simulink model "angleClosedloop_hw"  (R2020a)
settings: Solver=FixedStepAuto  StartTime=0.0  StopTime=30  FixedStep=TS  RelTol=1e-3  EnableMultiTasking=on
PostLoadFcn:
  | paramsBasicKinematics
  | load('MotorResponse.mat')
model workspace (MAT data in the model file):
  TS = 0.01
undefined symbols (not defined in the file): L, PWMcmdMono_L, PWMcmdMono_R, r, sigbuilder_block, speedMono_L, speedMono_R
libraries: arduinomotorcarrierlib x4, simulink_extras x4, simulink x1
settings Model: SimulationMode=external  SILPILModeSetting=veronly  ExtModeTrigDuration=2  Creator=jmodiset  LastModifiedBy=mmarathe
settings DataIOCC: ReturnWorkspaceOutputs=off
settings OptimizationCC: PassReuseOutputArgsThreshold=0  MaxStackSize=64
settings DebuggingCC: ParameterTunabilityLossMsg=error  PregeneratedLibrarySubsystemCodeDiagnostic=none  ArithmeticOperatorsInVariantConditions=warning
settings HardwareCC: ProdBitPerPointer=32  ProdBitPerSizeT=32  ProdBitPerPtrDiffT=32  ProdLargestAtomicInteger=Long  ProdLargestAtomicFloat=Double  ProdWordSize=32  ProdHWDeviceType=ARM Compatible->ARM Cortex
settings SFSimCC: SimUseLocalCustomCode=off  MATLABDynamicMemAlloc=off  CustomCodeUndefinedFunction=UseInterfaceOnly
settings RTWCC: SystemTargetFile=ert.tlc  HardwareBoard=Arduino Nano 33 IoT  TLCOptions=-aInlineSetEventsForThisBaseRateFcn=TLC_FALSE -aSuppressMultiTaskScheduler=TLC_FALSE -aRateBasedStepFcn=1  TemplateMakefile=ert_default_tmf  RTWUseLocalCustomCode=off  Toolchain=Arduino ARM  BuildConfiguration=Faster Runs
settings CodeAppCC: ForceParamTrailComments=on  OperatorAnnotations=on
settings ERTTargetCC: ERTCustomFileBanners=off  SupportContinuousTime=on  SupportNonInlinedSFcns=on  RemoveResetFunc=off  SupportVariableSizeSignals=on  ModelStepFunctionPrototypeControlCompliant=off  ExtModeStaticAllocSize=8192

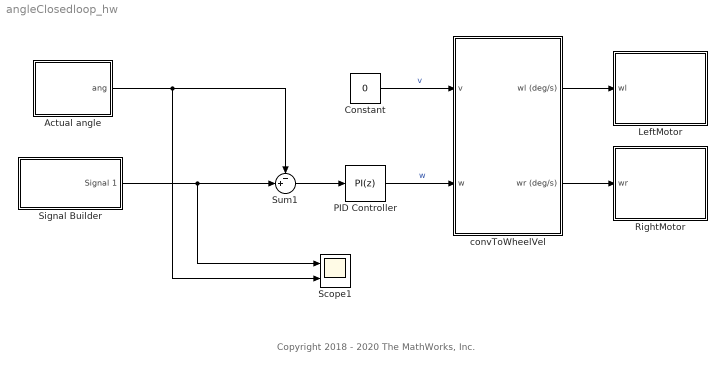
== system angleClosedloop_hw ==
  note: Copyright 2018 - 2020 The MathWorks, Inc.
  Actual angle : Subsystem
  Constant : Constant  Value=0
  LeftMotor : Subsystem
      mask Display:
      | color('white');
      | plot([100,100,100,100]*1,[100,100,100,100]*1);
      | plot([100,100,100,100]*0,[100,100,100,100]*0);
      | sppkgroot = strrep(codertarget.arduinobase.internal.getBaseSpPkgRootDir(),'\','/');
      | image(fullfile(sppkgroot,'resources','dcmotor.png'),'center')
  "PID Controller " : simulink/Continuous/PID Controller  Controller=PI  Form=Parallel  TimeDomain=Discrete-time  UseExternalTs=off  SampleTime=-1  IntegratorMethod=Forward Euler  FilterMethod=Forward Euler  ControllerParametersSource=internal  P=3  I=1  D=0  UseFilter=on  N=100  TunerSelectOption=Transfer Function Based (PID Tuner App)  InitialConditionSource=internal  InitialConditionForIntegrator=0  InitialConditionForFilter=0  DifferentiatorICPrevScaledInput=0  ExternalReset=none  TrackingMode=off  Kt=1  LimitOutput=off  UpperSaturationLimit=inf  LowerSaturationLimit=-inf  LinearizeAsGain=on  AntiWindupMode=none  Kb=1  POutMin=[]  POutMax=[]  IOutMin=[]  IOutMax=[]  DOutMin=[]  DOutMax=[]  NOutMin=[]  NOutMax=[]  SumOutMin=[]  SumOutMax=[]  SaturationOutMin=[]  SaturationOutMax=[]  PParamMin=[]  PParamMax=[]  IParamMin=[]  IParamMax=[]  DParamMin=[]  DParamMax=[]  NParamMin=[]  NParamMax=[]  KbParamMin=[]  KbParamMax=[]  KtParamMin=[]  KtParamMax=[]  KbOutMin=[]  KbOutMax=[]  KtOutMin=[]  KtOutMax=[]  IntegratorOutMin=[]  IntegratorOutMax=[]  FilterOutMin=[]  FilterOutMax=[]  SumI1OutMin=[]  SumI1OutMax=[]  SumI2OutMin=[]  SumI2OutMax=[]  SumI3OutMin=[]  SumI3OutMax=[]  SumI4OutMin=[]  SumI4OutMax=[]  SumDOutMin=[]  SumDOutMax=[]  DifferentiatorOutMin=[]  DifferentiatorOutMax=[]  FilterDiffOutCoefMin=[]  FilterDiffOutCoefMax=[]  ReciprocalOutMin=[]  ReciprocalOutMax=[]  SumDenOutMin=[]  SumDenOutMax=[]  SumNumOutMin=[]  SumNumOutMax=[]  DivideOutMin=[]  DivideOutMax=[]  UdiffTsProdOutMin=[]  UdiffTsProdOutMax=[]  NTsProdOutMin=[]  NTsProdOutMax=[]  UintegralTsProdOutMin=[]  UintegralTsProdOutMax=[]  UngainTsProdOutMin=[]  UngainTsProdOutMax=[]  IntegratorContinuousStateAttributes=''  IntegratorStateMustResolveToSignalObject=off  IntegratorRTWStateStorageClass=Auto  FilterContinuousStateAttributes=''  FilterStateMustResolveToSignalObject=off  FilterRTWStateStorageClass=Auto  ParallelPVariant=InternalParameters  IdealPVariant=Disabled  IVariant=InternalParameters  DVariant=Disabled  IntegratorVariant=Discrete  SatVariant=Disabled  AWVariant=Passthrough  PCopyVariant=Disabled  TRVariant=Disabled  FdbkBlocksVariant=Forward  IdealPFdbkVariant=Disabled  SatFdbkVariant=Disabled  DerivativeFilterVariant=Disabled  NVariant=Disabled  NCopyVariant=Disabled_SignalSpec  FilterICVariant=Disabled  IntegratorICVariant=InternalICs  ExternalResetVariant=Disabled  TRSumVariant=Passthrough  SumFdbkVariant=Disabled  SumVariant=Sum_PI  TsampFilterVariant=InternalTs  TsampNgainVariant=Passthrough  TsampIntegralVariant=Passthrough
  RightMotor : Subsystem
      mask Display:
      | color('white');
      | plot([100,100,100,100]*1,[100,100,100,100]*1);
      | plot([100,100,100,100]*0,[100,100,100,100]*0);
      | sppkgroot = strrep(codertarget.arduinobase.internal.getBaseSpPkgRootDir(),'\','/');
      | image(fullfile(sppkgroot,'resources','dcmotor.png'),'center')
  Scope1 : Scope  NumInputPorts=2
  "Signal Builder " : Subsystem  Tag=STV Subsys  LoadFcn=sigbuilder_block('load');  StartFcn=sigbuilder_block('start');  StopFcn=sigbuilder_block('stop');  ClipboardFcn=sigbuilder_block('clipboard');  mask(Sigbuilder block){tuvar=[0:10]}
      mask help: Simulink:masks:SigbuilderBlock_MD
      mask init:
      | if ~strcmp(get_param(bdroot(gcbh),'SimulationStatus'),'stopped') tuvar = sigbuilder_block('maskInit'); end
      settings: CopyFcn=sigbuilder_block('copy');  DeleteFcn=sigbuilder_block('delete');  ModelCloseFcn=sigbuilder_block('modelClose');  PreSaveFcn=sigbuilder_block('preSave');  PauseFcn=sigbuilder_block('pause');  ContinueFcn=sigbuilder_block('continue');  NameChangeFcn=sigbuilder_block('namechange');  OpenFcn=sigbuilder_block('open',[256.5 124.5 550.5 399.75 ]);  CloseFcn=sigbuilder_block('close');
      mask Display: plot(0, 0, 100, 100,[2, 2, 32, 32, 2], [68, 8, 8, 68, 68],[32, 2], [38, 38], [32, 19, 2],[53, 60, 44], [32, 17, 17, 2],[16, 16, 31, 31]);txt = getActiveGroup(gcbh);text(2, 100, txt,'verticalAlignment', 'top');
  Sum1 : Sum  Inputs=-+|
  convToWheelVel : Subsystem
  wires:
  Actual angle/1(ang) -> Scope1/2, Sum1/1
  Sum1/1 -> "PID Controller "/1
  "Signal Builder "/1(Signal 1) -> Sum1/2, Scope1/1
  Constant/1 -> convToWheelVel/1(v)  "v"
  "PID Controller "/1 -> convToWheelVel/2(w)  "w"
  convToWheelVel/1(wl (deg/s)) -> LeftMotor/1(wl)
  convToWheelVel/2(wr (deg/s)) -> RightMotor/1(wr)

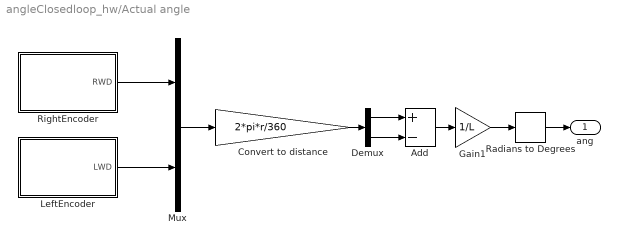
== system angleClosedloop_hw/Actual angle ==
  Add : Sum  Inputs=+-
  Convert to distance : Gain  Gain=2*pi*r/360
  Demux : Demux  Outputs=2
  Gain1 : Gain  Gain=1/L
  LeftEncoder : Subsystem
  Mux : Mux  Inputs=2
  Radians to Degrees : simulink_extras/Transformations/Radians to Degrees
  RightEncoder : Subsystem
  ang : Outport  VectorParamsAs1DForOutWhenUnconnected=off
  wires:
  RightEncoder/1(RWD) -> Mux/1
  Gain1/1 -> Radians to Degrees/1
  Add/1 -> Gain1/1
  Demux/2 -> Add/2
  Convert to distance/1 -> Demux/1
  Demux/1 -> Add/1
  Mux/1 -> Convert to distance/1
  LeftEncoder/1(LWD) -> Mux/2
  Radians to Degrees/1 -> ang/1

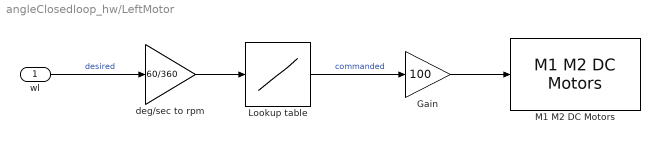
== system angleClosedloop_hw/LeftMotor ==
  wl : Inport
  Gain : Gain  Gain=100
  Lookup table : Lookup_n-D  NumberOfTableDimensions=1  BreakpointsForDimension1=speedMono_L  Table=PWMcmdMono_L  UseLastTableValue=on  InternalRulePriority=Speed  RndMeth=Simplest  InputSameDT=on
  M1 M2 DC Motors : arduinomotorcarrierlib/M1 M2 DC Motors  SlaveAddress=uint8( hex2dec( '66' ) )  blockPlatform=ARDUINO  MotorNumber=M2  MotorCarrierPWMFreq=100
      settings: SourceProductName=Simulink Support Package for Arduino Hardware
  deg/sec to rpm : Gain  Gain=60/360
  wires:
  wl/1 -> deg/sec to rpm/1  "desired"
  Lookup table/1 -> Gain/1  "commanded"
  Gain/1 -> M1 M2 DC Motors/1
  deg/sec to rpm/1 -> Lookup table/1

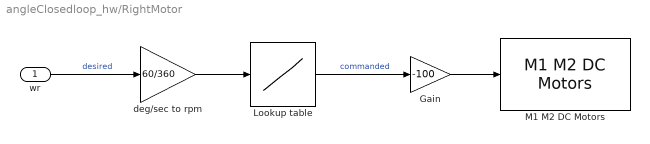
== system angleClosedloop_hw/RightMotor ==
  wr : Inport
  Gain : Gain  Gain=-100
  Lookup table : Lookup_n-D  NumberOfTableDimensions=1  BreakpointsForDimension1=speedMono_R  Table=PWMcmdMono_R  UseLastTableValue=on  InternalRulePriority=Speed  RndMeth=Simplest  InputSameDT=on
  M1 M2 DC Motors : arduinomotorcarrierlib/M1 M2 DC Motors  SlaveAddress=uint8( hex2dec( '66' ) )  blockPlatform=ARDUINO  MotorNumber=M1  MotorCarrierPWMFreq=100
      settings: SourceProductName=Simulink Support Package for Arduino Hardware
  deg/sec to rpm : Gain  Gain=60/360
  wires:
  wr/1 -> deg/sec to rpm/1  "desired"
  Lookup table/1 -> Gain/1  "commanded"
  Gain/1 -> M1 M2 DC Motors/1
  deg/sec to rpm/1 -> Lookup table/1

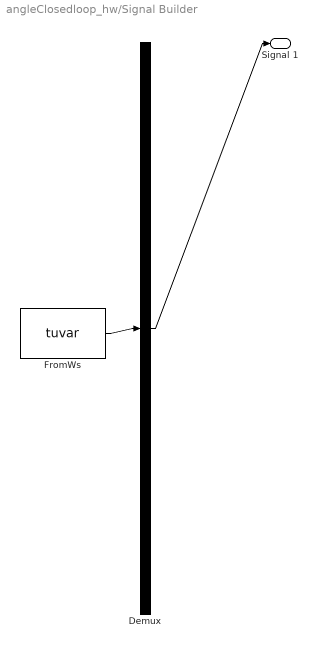
== system angleClosedloop_hw/Signal Builder  ==
  Demux : Demux  Tag=STV Demux  Outputs=1
      settings: DisplayOption=none
  FromWs : FromWorkspace  Tag=STV FromWs  VariableName=tuvar
      SigBuilderData=|
      | common.afterFinalStr = 'Extrapolate'
      | common.sampleTime = 0
      | dataSet.timeRange = [0 30]
      | dataSet.name = 'Group 1'
      | sbobj.Groups.Name = 'Group 1'
      | sbobj.Groups.Signals.Name = 'Signal 1'
      | sbobj.Groups.Signals.XData = [0 5 5 30]
      | sbobj.Groups.Signals.YData = [0 0 90 90]
      | sbobj.Groups.TimeRange = [0 30]
  Signal 1 : Outport  Tag=STV Outport  VectorParamsAs1DForOutWhenUnconnected=off
  wires:
  Demux/1 -> Signal 1/1
  FromWs/1 -> Demux/1

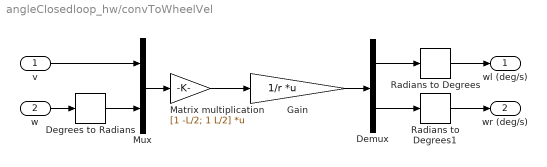
== system angleClosedloop_hw/convToWheelVel ==
  v : Inport
  w : Inport  Port=2
  " Gain" : Gain  Gain=1/r  Multiplication=Matrix(K*u)
  Degrees to Radians : simulink_extras/Transformations/Degrees to Radians
  Demux : Demux  Outputs=2
  Matrix multiplication : Gain  Gain=[1 -L/2; 1 L/2]  Multiplication=Matrix(K*u)
  Mux : Mux  Inputs=2
  Radians to Degrees : simulink_extras/Transformations/Radians to Degrees
  Radians to Degrees1 : simulink_extras/Transformations/Radians to Degrees
  wl (deg/s) : Outport  VectorParamsAs1DForOutWhenUnconnected=off
  wr (deg/s) : Outport  Port=2  VectorParamsAs1DForOutWhenUnconnected=off
  wires:
  " Gain"/1 -> Demux/1
  Matrix multiplication/1 -> " Gain"/1
  v/1 -> Mux/1
  Mux/1 -> Matrix multiplication/1
  Demux/1 -> Radians to Degrees/1
  Demux/2 -> Radians to Degrees1/1
  w/1 -> Degrees to Radians/1
  Radians to Degrees/1 -> wl (deg/s)/1
  Radians to Degrees1/1 -> wr (deg/s)/1
  Degrees to Radians/1 -> Mux/2

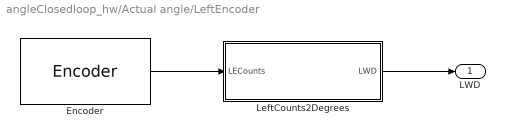
== system angleClosedloop_hw/Actual angle/LeftEncoder ==
  Encoder : arduinomotorcarrierlib/Encoder  SlaveAddress=uint8( hex2dec( '66' ) )  blockPlatform=ARDUINO  Encoder=2  ShowSpeed=off  ResetOption=on  SampleTime=0.01
      settings: SourceProductBaseCode=ARDUINO
  LeftCounts2Degrees : Subsystem
  LWD : Outport  VectorParamsAs1DForOutWhenUnconnected=off
  wires:
  LeftCounts2Degrees/1(LWD) -> LWD/1
  Encoder/1 -> LeftCounts2Degrees/1(LECounts)

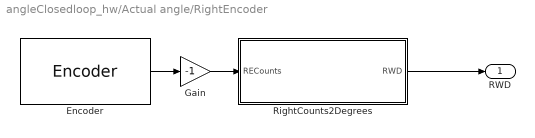
== system angleClosedloop_hw/Actual angle/RightEncoder ==
  Encoder : arduinomotorcarrierlib/Encoder  SlaveAddress=uint8( hex2dec( '66' ) )  blockPlatform=ARDUINO  Encoder=1  ShowSpeed=off  ResetOption=on  SampleTime=0.01
      settings: SourceProductBaseCode=ARDUINO
  Gain : Gain  Gain=-1
  RightCounts2Degrees : Subsystem
  RWD : Outport  VectorParamsAs1DForOutWhenUnconnected=off
  wires:
  RightCounts2Degrees/1(RWD) -> RWD/1
  Encoder/1 -> Gain/1
  Gain/1 -> RightCounts2Degrees/1(RECounts)

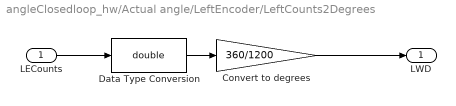
== system angleClosedloop_hw/Actual angle/LeftEncoder/LeftCounts2Degrees ==
  LECounts : Inport
  Convert to degrees : Gain  Gain=360/1200
  Data Type Conversion : DataTypeConversion  OutDataTypeStr=double
  LWD : Outport  VectorParamsAs1DForOutWhenUnconnected=off
  wires:
  LECounts/1 -> Data Type Conversion/1
  Data Type Conversion/1 -> Convert to degrees/1
  Convert to degrees/1 -> LWD/1

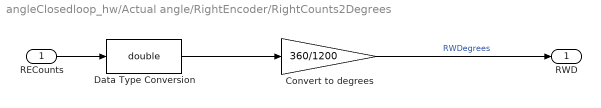
== system angleClosedloop_hw/Actual angle/RightEncoder/RightCounts2Degrees ==
  RECounts : Inport
  Convert to degrees : Gain  Gain=360/1200
  Data Type Conversion : DataTypeConversion  OutDataTypeStr=double
  RWD : Outport  VectorParamsAs1DForOutWhenUnconnected=off
  wires:
  Data Type Conversion/1 -> Convert to degrees/1
  RECounts/1 -> Data Type Conversion/1
  Convert to degrees/1 -> RWD/1  "RWDegrees"
